simulink model "Video"  (R2021a)
settings: Solver=FixedStepDiscrete  StartTime=0.0  StopTime=20  RelTol=1e-3  EnableMultiTasking=on
undefined symbols (not defined in the file): gray, Rec, SDTV
libraries: visionconversions x3, visionstatistics x2, dspvision x2, dspstat3 x2
settings Model: Creator=leszczuk  LastModifiedBy=miklesz
settings SolverCC: AlgebraicLoopSolver=TrustRegion
settings DataIOCC: LimitDataPoints=on  SaveFormat=Array  SignalLoggingSaveFormat=ModelDataLogs  ReturnWorkspaceOutputs=off
settings OptimizationCC: ExpressionDepthLimit=2147483647  InitFltsAndDblsToZero=on  LifeSpan=inf
settings DebuggingCC: SaveWithParameterizedLinksMsg=none  UnderspecifiedInitializationDetection=Classic  MergeDetectMultiDrivingBlocksExec=none  SolverPrmCheckMsg=warning  FcnCallInpInsideContextMsg=warning  StateNameClashWarn=warning  SFUnexpectedBacktrackingDiag=warning  SFNoUnconditionalDefaultTransitionDiag=warning  SFMachineParentedDataDiag=warning  ArithmeticOperatorsInVariantConditions=warning
settings HardwareCC: ProdBitPerPointer=32  ProdBitPerSizeT=32  ProdBitPerPtrDiffT=32  ProdLargestAtomicFloat=None  ProdIntDivRoundTo=Undefined  ProdEndianess=Unspecified  ProdWordSize=32  ProdHWDeviceType=32-bit Generic
settings ModelReferenceCC: PropagateSignalLabelsOutOfModel=off
settings SFSimCC: SimUseLocalCustomCode=off  CustomCodeUndefinedFunction=UseInterfaceOnly
settings RTWCC: RTWUseLocalCustomCode=off
settings CodeAppCC: StateflowObjectComments=on
settings GRTTargetCC: TargetFcnLib=ansi_tfl_tmw.mat  TargetLangStandard=C89/C90 (ANSI)  CombineOutputUpdateFcns=off  GRTInterface=on
settings ConfigComp: CovMetricSettings=dw  CovSaveCumulativeToWorkspaceVar=on  CovSaveSingleToWorkspaceVar=on  CovExternalEMLEnable=off

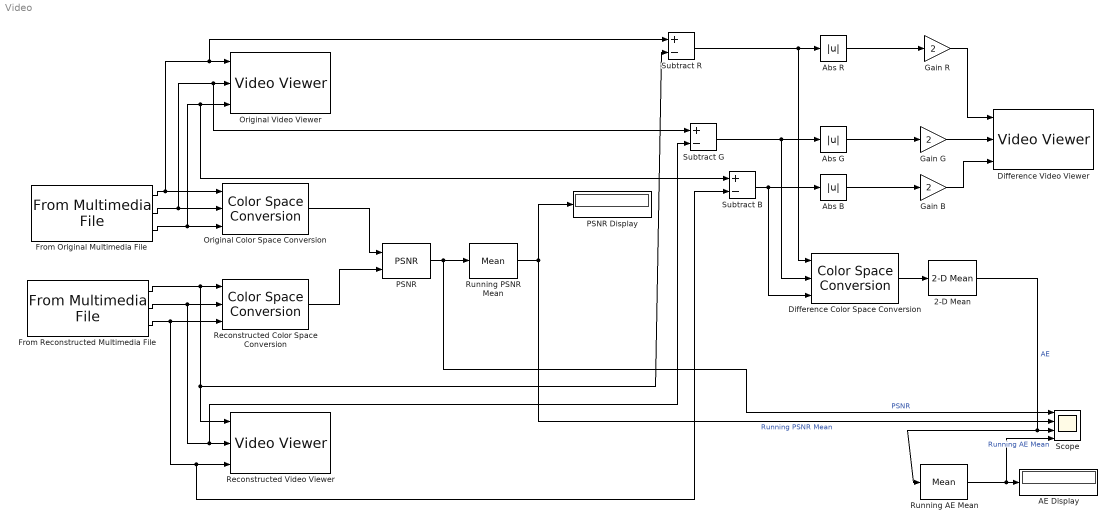
== system Video ==
  2-D Mean : visionstatistics/2-D Mean  run=off  reset_popup=None  directionMode=Entire input  dimension=1  treatSBRowAsCol=on  outputLastDataTypeStr=Inherit: Same as accumulator  accumMode=Binary point scaling  accumWordLength=32  accumFracLength=0  accumLastDataTypeStr=fixdt([],32,0)  roiEnable=off  roiType=Rectangles  roiPortion=Entire ROI  roiOutput=Individual statistics for each ROI  roiFlag=off  roundingMode=Floor  overflowMode=off  accumDataTypeStr=fixdt([],32,0)  outputDataTypeStr=Inherit: Same as accumulator  outputMin=[]  outputMax=[]
      settings: SourceProductBaseCode=VP
  AE Display : Display
  Abs B : Abs
  Abs G : Abs
  Abs R : Abs
  Difference Color Space Conversion : visionconversions/Color Space  Conversion  conversion=Obsolete  conversionActive=R'G'B' to intensity  wp_str=D65  rec=Rec. 601 (SDTV)  sys=1125/60/2:1  imagePorts=Separate color signals
  Difference Video Viewer : VideoViewer  imagePorts=separate color signals  colormapValue=gray(256)  FigPos=[552 383 176 144]  AxisZoom=off  trueSizedOnce=on
  From Original Multimedia File : dspvision/From Multimedia File  inputFilename=/Users/miklesz/OneDrive - Akademia Górniczo-Hutnicza im. Stanisława Staszica w Krakowie/Documents/AGH/Teaching/Courses/Multimedia Information Processing and Communications/Topics/agh_src1_hrc0.m4v  readRange=[1 Inf]  loop=on  numPlays=1  outputStreams=Video only  videoDataType=single  audioDataType=int16  inheritSampleTime=on  userDefinedSampleTime=1/30  noAudioOutput=off  isIntensityVideo=off  fourcc=RGB  colorVideoFormat=Separate color signals  outputEOF=off  dataOrg=Column-major  audioFrameSize=1024  computeAudioFrameSize=off  outSamplingMode=Frame based
  From Reconstructed Multimedia File : dspvision/From Multimedia File  inputFilename=/Users/miklesz/OneDrive - Akademia Górniczo-Hutnicza im. Stanisława Staszica w Krakowie/Documents/AGH/Teaching/Courses/Multimedia Information Processing and Communications/Topics/agh_src1_hrc_h264.mp4  readRange=[1 Inf]  loop=on  numPlays=1  outputStreams=Video only  videoDataType=single  audioDataType=int16  inheritSampleTime=on  userDefinedSampleTime=1/30  noAudioOutput=off  isIntensityVideo=off  fourcc=RGB  colorVideoFormat=Separate color signals  outputEOF=off  dataOrg=Column-major  audioFrameSize=1024  computeAudioFrameSize=off  outSamplingMode=Frame based
  Gain B : Gain  Gain=2
  Gain G : Gain  Gain=2
  Gain R : Gain  Gain=2
  Original Color Space Conversion : visionconversions/Color Space  Conversion  conversion=Obsolete  conversionActive=R'G'B' to intensity  wp_str=D65  rec=Rec. 601 (SDTV)  sys=1125/60/2:1  imagePorts=Separate color signals
  Original Video Viewer : VideoViewer  imagePorts=separate color signals  colormapValue=gray(256)  FigPos=[552 383 176 144]  AxisZoom=off  trueSizedOnce=on
  PSNR : visionstatistics/PSNR
      settings: SourceProductBaseCode=VP
  PSNR Display : Display
  Reconstructed Color Space Conversion : visionconversions/Color Space  Conversion  conversion=Obsolete  conversionActive=R'G'B' to intensity  wp_str=D65  rec=Rec. 601 (SDTV)  sys=1125/60/2:1  imagePorts=Separate color signals
  Reconstructed Video Viewer : VideoViewer  imagePorts=separate color signals  colormapValue=gray(256)  FigPos=[552 383 176 144]  AxisZoom=off  trueSizedOnce=on
  Running AE Mean : dspstat3/Mean  run=on  InputProcessing=Columns as channels (frame based)  reset_popup=None  directionMode=Each column  dimension=1  roiEnable=off  roiType=Rectangles  roiPortion=Entire ROI  roiOutput=Individual statistics for each ROI  roiFlag=off  roundingMode=Floor  overflowMode=off  outputDataTypeStr=Inherit: Same as accumulator  outputMin=[]  outputMax=[]  outputLastDataTypeStr=Inherit: Same as accumulator
  Running PSNR Mean : dspstat3/Mean  run=on  InputProcessing=Columns as channels (frame based)  reset_popup=None  directionMode=Each column  dimension=1  roiEnable=off  roiType=Rectangles  roiPortion=Entire ROI  roiOutput=Individual statistics for each ROI  roiFlag=off  roundingMode=Floor  overflowMode=off  outputDataTypeStr=Inherit: Same as accumulator  outputMin=[]  outputMax=[]  outputLastDataTypeStr=Inherit: Same as accumulator
  Scope : Scope  NumInputPorts=4
  Subtract B : Sum  Inputs=+-
  Subtract G : Sum  Inputs=+-
  Subtract R : Sum  Inputs=+-
  wires:
  PSNR/1 -> Running PSNR Mean/1, Scope/1  "PSNR"
  From Original Multimedia File/1 -> Original Color Space Conversion/1, Original Video Viewer/1, Subtract R/1
  From Reconstructed Multimedia File/1 -> Reconstructed Color Space Conversion/1, Reconstructed Video Viewer/1, Subtract R/2
  Original Color Space Conversion/1 -> PSNR/1
  Reconstructed Color Space Conversion/1 -> PSNR/2
  From Original Multimedia File/2 -> Original Color Space Conversion/2, Original Video Viewer/2, Subtract G/1
  From Original Multimedia File/3 -> Original Color Space Conversion/3, Original Video Viewer/3, Subtract B/1
  From Reconstructed Multimedia File/2 -> Reconstructed Color Space Conversion/2, Reconstructed Video Viewer/2, Subtract G/2
  From Reconstructed Multimedia File/3 -> Reconstructed Color Space Conversion/3, Reconstructed Video Viewer/3, Subtract B/2
  Subtract B/1 -> Abs B/1, Difference Color Space Conversion/3
  Subtract G/1 -> Abs G/1, Difference Color Space Conversion/2
  Subtract R/1 -> Abs R/1, Difference Color Space Conversion/1
  Abs R/1 -> Gain R/1
  Abs G/1 -> Gain G/1
  Abs B/1 -> Gain B/1
  Gain R/1 -> Difference Video Viewer/1
  Gain G/1 -> Difference Video Viewer/2
  Gain B/1 -> Difference Video Viewer/3
  Difference Color Space Conversion/1 -> 2-D Mean/1
  Running PSNR Mean/1 -> PSNR Display/1, Scope/2  "Running PSNR Mean"
  2-D Mean/1 -> Scope/3, Running AE Mean/1  "AE"
  Running AE Mean/1 -> Scope/4, AE Display/1  "Running AE Mean"
